simulink subsystem "rss_MotoSTMSenl"  (R2023a)
settings: Solver=VariableStepAuto  StartTime=0.0  StopTime=10.0  RelTol=1e-3
undefined symbols (not defined in the file): Cdbl_nElecAgSpdMaxVal, Gs16_nMinSenlRefElecSpd_C, Gs16_nOpnLpConvActElecSpd_C, Gs16_nShOffActElecSpd_C
settings Model: Creator=xiaoqiang.yuan  LastModifiedBy=xiaoqiang.yuan

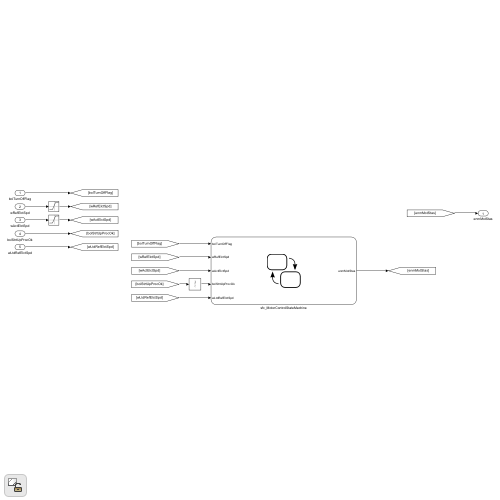
[thumbnail: Simulink's stored preview of the top-level diagram]
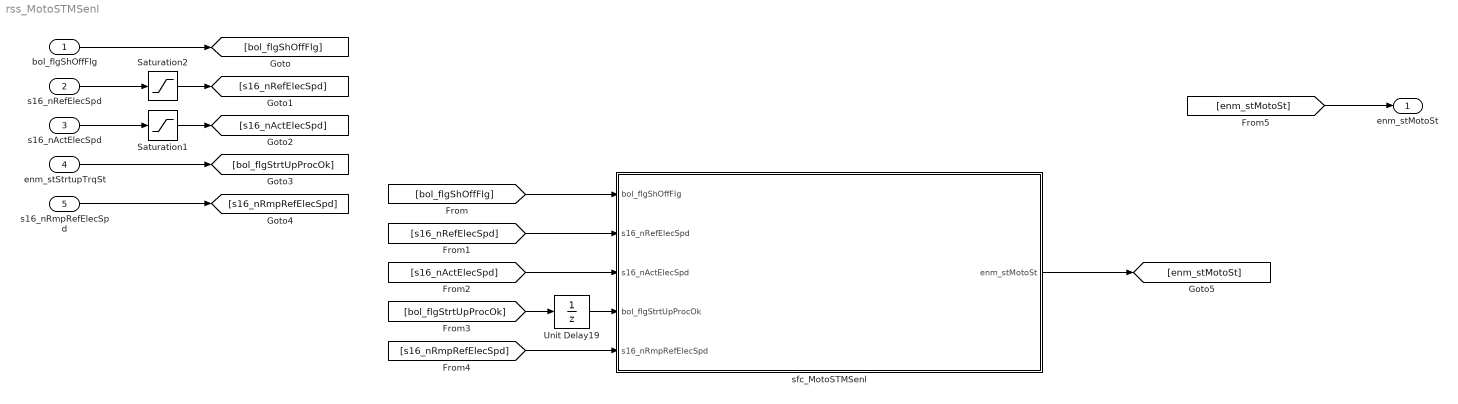
== system rss_MotoSTMSenl ==
  bol_flgShOffFlg : Inport  OutDataTypeStr=boolean
  s16_nRefElecSpd : Inport  Port=2  OutDataTypeStr=dt_Standardize_s16p15b0
  s16_nActElecSpd : Inport  Port=3  OutDataTypeStr=dt_Standardize_s16p15b0
  enm_stStrtupTrqSt : Inport  Port=4  OutDataTypeStr=boolean
  s16_nRmpRefElecSpd : Inport  Port=5  OutDataTypeStr=dt_Standardize_s16p15b0
  Saturation1 : Saturate  UpperLimit=Cdbl_nElecAgSpdMaxVal  LowerLimit=-Cdbl_nElecAgSpdMaxVal
  Saturation2 : Saturate  UpperLimit=Cdbl_nElecAgSpdMaxVal  LowerLimit=-Cdbl_nElecAgSpdMaxVal
  Unit Delay19 : UnitDelay  SampleTime=-1  HasFrameUpgradeWarning=on
  sfc_MotoSTMSenl : Stateflow chart  TreatAsAtomicUnit=on
  enm_stMotoSt : Outport  OutDataTypeStr=Enum: ENM_MOTO_STATUS
  wires:
  Unit Delay19/1 -> sfc_MotoSTMSenl/4(bol_flgStrtUpProcOk)
  enm_stStrtupTrqSt/1 -> [bol_flgStrtUpProcOk]
  bol_flgShOffFlg/1 -> [bol_flgShOffFlg]
  s16_nActElecSpd/1 -> Saturation1/1
  Saturation2/1 -> [s16_nRefElecSpd]
  Saturation1/1 -> [s16_nActElecSpd]
  s16_nRefElecSpd/1 -> Saturation2/1
  s16_nRmpRefElecSpd/1 -> [s16_nRmpRefElecSpd]
  [bol_flgShOffFlg] -> sfc_MotoSTMSenl/1(bol_flgShOffFlg)
  [s16_nRefElecSpd] -> sfc_MotoSTMSenl/2(s16_nRefElecSpd)
  [s16_nActElecSpd] -> sfc_MotoSTMSenl/3(s16_nActElecSpd)
  [bol_flgStrtUpProcOk] -> Unit Delay19/1
  [s16_nRmpRefElecSpd] -> sfc_MotoSTMSenl/5(s16_nRmpRefElecSpd)
  sfc_MotoSTMSenl/1(enm_stMotoSt) -> [enm_stMotoSt]
  [enm_stMotoSt] -> enm_stMotoSt/1

== stateflow chart rss_MotoSTMSenl/sfc_MotoSTMSenl ==
  state OFF
    en:
    enm_stMotoSt = ENM_MOTO_STATUS.OFF;
  state CLOSED_LOOP
    en:
    enm_stMotoSt = ENM_MOTO_STATUS.CLOSED_LOOP;
  state OPEN_LOOP
    en:
    enm_stMotoSt = ENM_MOTO_STATUS.OPEN_LOOP;
  (default) -> OFF
  (junction 29) -> OFF
  (junction 14) -> OFF
  OPEN_LOOP -> (junction 29) [order 2] : [(s16_nRefElecSpd == 0 && ...
      | abs(s16_nActElecSpd) < abs(Gs16_nShOffActElecSpd_C)) || ...
      | bol_flgShOffFlg]
  CLOSED_LOOP -> (junction 14) [order 1] : [(s16_nRefElecSpd == 0 && ...
      | abs(s16_nActElecSpd) < abs(Gs16_nShOffActElecSpd_C)) || ...
      | bol_flgShOffFlg]
  OFF -> (junction 6) : [abs(s16_nRefElecSpd) > 0 && ...
      | not(bol_flgShOffFlg)]
  (junction 6) -> OPEN_LOOP
  OPEN_LOOP -> CLOSED_LOOP [order 1] : [s16_nRefElecSpd ~= 0 && bol_flgStrtUpProcOk && abs(s16_nRmpRefElecSpd) >= abs(Gs16_nMinSenlRefElecSpd_C)]
  CLOSED_LOOP -> OPEN_LOOP [order 2] : [s16_nRefElecSpd ~= 0 && abs(s16_nRmpRefElecSpd) < abs(Gs16_nMinSenlRefElecSpd_C) &&...
      |  abs(s16_nActElecSpd) < abs(Gs16_nOpnLpConvActElecSpd_C)]
  data: Gs16_nShOffActElecSpd_C parameter; Gs16_nMinSenlRefElecSpd_C parameter; Gs16_nOpnLpConvActElecSpd_C parameter; bol_flgShOffFlg input boolean; s16_nRefElecSpd input dt_Standardize_s16p15b0; s16_nActElecSpd input dt_Standardize_s16p15b0; enm_stMotoSt output Enum: ENM_MOTO_STATUS; bol_flgStrtUpProcOk input boolean; s16_nRmpRefElecSpd input dt_Standardize_s16p15b0
